simulink model "AirRefueling_Platform_ch10_WindEffect"  (R2022a)
settings: Solver=ode3  StartTime=0.0  StopTime=150  FixedStep=0.01  RelTol=1e-5  AbsTol=1e-4  EnableMultiTasking=on
InitFcn:
  | F16_Init
values from neighbouring files (symbols this model uses):
  airSpeed = 393.72    [F16_Init.m]
  alpha0 = trimAlpha*180/pi    (= 6.62393794015)    [F16_Init.m]
  altitude = 9843    [F16_Init.m]
  b_ref = 30.0    (= 30)    [F16_Init.m]
  C = [ 1,0,0,zeros(1,15) ... (first row only)    [F16_Init.m]
  C2m = [C(1,:) ... (first row only)    [F16_Init.m]
  d_f_rc = [4.45;0;-3.81]    [F16_Init.m]
  d_pr_rc = [8.2;0.45;-3.3]    [F16_Init.m]
  dLEF = 0    [F16_Init.m]
  fi_flag = 1    [F16_Init.m]
  Kc = [ ... (first row only)    [F16_Init.m]
  Ki = zeros(4,3)    [F16_Init.m]
  Kp = zeros(4,18)    [F16_Init.m]
  mass = 636.94    [F16_Init.m]
  p0_pr = p0_rc + d_pr_rc    [F16_Init.m]
  p0_rc = [-28;0;0]    [F16_Init.m]
  trim_ail = 0.00874607850103852    (= 0.00874607850104)    [F16_Init.m]
  trim_control = [trim_thrust;trim_ele;trim_ail;trim_rud]    [F16_Init.m]
  trim_ele = -2.97973164860638    (= -2.97973164861)    [F16_Init.m]
  trim_rud = 0.0680302158182712    (= 0.0680302158183)    [F16_Init.m]
  trim_state1 = [trim_state;0;0;0;0;0;0]    [F16_Init.m]
  trim_thrust = 2279.08519954656    (= 2279.08519955)    [F16_Init.m]
  visual_err = [0;0;0]    [F16_Init.m]
undefined symbols (not defined in the file or in its folder): Cdr_, dockingPoint, dtheta10, dtheta20, F, height, k_reel, kd, l0, l1, l_density, Light, m0, Mdr, MIL, N, Rdr, Rl, STD, T_reel_initial, theta10, theta20, vt0
libraries: etargetslib x22, dspnetwork x20, aerolibconvert2 x6, aerolibasang x4, simulink x2, aerolibatmos2 x2, aerolibwind2 x2, aerolibobsolete x2, sharedtransform x2, aerolibutil x2, vrlib x1, aerolibadyn x1
(part 2 of 4)

== system AirRefueling_Platform_ch10_WindEffect/3D rendering engine/SendToPX4SILIntFloat ==
  note: struct PX4SILIntFloat {
      | int checksum ;
      | int CopterID ;
      | int inSILInts [ 8 ];
      | float inSILFLoats [ 20 ];
      | }
  note: This message will be sent to PX4 DLL model's input signals inSILInts[8] and inSILFloats[20].
      | The checksum should be set to 1234567897, and the data should be sent to port 30100+(i-1)*2
  inSILInts : Inport  OutDataTypeStr=int32  PortDimensions=8
  inSILFloats : Inport  Port=2  OutDataTypeStr=single  PortDimensions=20
  CopterID : Constant  Value=10  OutDataTypeStr=Inherit: Inherit via back propagation
  Data Type Conversion1 : DataTypeConversion  OutDataTypeStr=int32  SaturateOnIntegerOverflow=off  RndMeth=Floor
  Data Type Conversion2 : DataTypeConversion  OutDataTypeStr=single  SaturateOnIntegerOverflow=off  RndMeth=Floor
  Data Type Conversion3 : DataTypeConversion  OutDataTypeStr=int32  SaturateOnIntegerOverflow=off  RndMeth=Floor
  Mux : Mux  Inputs=2
  PayLoad : etargetslib/Byte Pack  datatypes={'int32','int32','single'}  byteAlign=8
  checksum : Constant  Value=1234567897  OutDataTypeStr=Inherit: Inherit via back propagation
  PX4SILIntFloat : Outport  OutDataTypeStr=uint8  PortDimensions=120  VectorParamsAs1DForOutWhenUnconnected=off
  wires:
  inSILFloats/1 -> Data Type Conversion2/1
  inSILInts/1 -> Data Type Conversion1/1
  PayLoad/1 -> PX4SILIntFloat/1
  Data Type Conversion1/1 -> PayLoad/2
  Data Type Conversion2/1 -> PayLoad/3
  checksum/1 -> Mux/1
  Mux/1 -> Data Type Conversion3/1
  Data Type Conversion3/1 -> PayLoad/1
  CopterID/1 -> Mux/2

== system AirRefueling_Platform_ch10_WindEffect/3D rendering engine/Subsystem1 ==
  copterID : Inport  PortDimensions=1
  vehicleType : Inport  Port=2  PortDimensions=1
  PosE : Inport  Port=3  PortDimensions=3
  AngEuler : Inport  Port=4  PortDimensions=3
  VelE : Inport  Port=5  PortDimensions=3
  Clock : Clock
  Constant1 : Constant  Value=[0,0,0,0]
  Constant3 : Constant  Value=[0,0,0]
  Constant4 : Constant  Value=[0,0,0]
  Constant5 : Constant  Value=[0,0,0]
  MotorPWMs1 : Constant  Value=[1000,1000,1000,1000,0,0,0,0]
  Subsystem : Subsystem
  toUnReal : Outport  VectorParamsAs1DForOutWhenUnconnected=off
  wires:
  VelE/1 -> Subsystem/4("VelE ")
  PosE/1 -> Subsystem/5(PosE)
  vehicleType/1 -> Subsystem/2(vehicleType)
  Clock/1 -> Subsystem/3(runnedTime)
  Constant4/1 -> Subsystem/10(RateB)
  Constant5/1 -> Subsystem/11(PosGPS)
  AngEuler/1 -> Subsystem/6(AngEuler)
  Subsystem/1(toUnReal) -> toUnReal/1
  Constant3/1 -> Subsystem/9(AccB)
  Constant1/1 -> Subsystem/7(AngQuatern)
  copterID/1 -> Subsystem/1(copterID)
  MotorPWMs1/1 -> Subsystem/8(MotorRPMS)

== system AirRefueling_Platform_ch10_WindEffect/3D rendering engine/VehicleAttatchreq ==
  note: struct VehicleAttatch25 {
      | 	int checksum;//1234567892
      | 	int CopterIDs[25];
      | 	int AttatchIDs[25];
      | 	int AttatchTypes[25];//0：正常模式，1：相对位置不相对姿态，2：相对位置+偏航（不相对俯仰和滚转），3：相对位置+全姿态（俯仰滚转偏航）
      | }
  CopterIDs : Inport  PortDimensions=25
  AttatchIDs : Inport  Port=2  PortDimensions=25
  AttatchTypes : Inport  Port=3  PortDimensions=25
  Constant7 : Constant  Value=1234567892
  Data Type Conversion{,1..2,4} (4 alike) : DataTypeConversion  OutDataTypeStr=int32  SaturateOnIntegerOverflow=off  RndMeth=Floor
  PayLoad : etargetslib/Byte Pack  datatypes={'int32','int32','int32','int32'}  byteAlign=4
  Out1 : Outport  VectorParamsAs1DForOutWhenUnconnected=off
  wires:
  Data Type Conversion1/1 -> PayLoad/3
  AttatchTypes/1 -> Data Type Conversion2/1
  Data Type Conversion2/1 -> PayLoad/4
  PayLoad/1 -> Out1/1
  AttatchIDs/1 -> Data Type Conversion1/1
  Data Type Conversion/1 -> PayLoad/2
  CopterIDs/1 -> Data Type Conversion/1
  Constant7/1 -> Data Type Conversion4/1
  Data Type Conversion4/1 -> PayLoad/1

== system AirRefueling_Platform_ch10_WindEffect/3D rendering engine1/20APIWithScale ==
  note: struct Multi3DData1New {
      |        int checksum;
      | 	uint16 IDs[20];
      | 	uint16 VehileTypes[20];
      | 	float PosE[60];
      | 	float AngEuler[60];
      | 	uint16 ScaleXYZ[60];
      | }
  note: scale value * 100
  IDs : Inport  PortDimensions=20
  VehileTypes : Inport  Port=2  PortDimensions=20
  PosEs : Inport  Port=3  PortDimensions=60
  AngEulers : Inport  Port=4  PortDimensions=60
  scaleXYZ : Inport  Port=5  PortDimensions=60
  Constant7 : Constant  Value=1234567890
  Data Type Conversion : DataTypeConversion  OutDataTypeStr=uint16  SaturateOnIntegerOverflow=off  RndMeth=Floor
  Data Type Conversion1 : DataTypeConversion  OutDataTypeStr=uint16  SaturateOnIntegerOverflow=off  RndMeth=Floor
  Data Type Conversion2 : DataTypeConversion  OutDataTypeStr=single  SaturateOnIntegerOverflow=off  RndMeth=Floor
  Data Type Conversion3 : DataTypeConversion  OutDataTypeStr=single  SaturateOnIntegerOverflow=off  RndMeth=Floor
  Data Type Conversion4 : DataTypeConversion  OutDataTypeStr=uint16  SaturateOnIntegerOverflow=off  RndMeth=Floor
  Data Type Conversion5 : DataTypeConversion  OutDataTypeStr=int32  SaturateOnIntegerOverflow=off  RndMeth=Floor
  Gain : Gain  Gain=100
  PayLoad : etargetslib/Byte Pack  datatypes={'int32','uint16','uint16','single','single','uint16'}  byteAlign=4
  Saturation : Saturate  UpperLimit=655.35  LowerLimit=0.01
  Out1 : Outport  VectorParamsAs1DForOutWhenUnconnected=off
  wires:
  Data Type Conversion3/1 -> PayLoad/5
  Data Type Conversion1/1 -> PayLoad/3
  PosEs/1 -> Data Type Conversion2/1
  Data Type Conversion2/1 -> PayLoad/4
  AngEulers/1 -> Data Type Conversion3/1
  PayLoad/1 -> Out1/1
  VehileTypes/1 -> Data Type Conversion1/1
  Data Type Conversion/1 -> PayLoad/2
  IDs/1 -> Data Type Conversion/1
  scaleXYZ/1 -> Saturation/1
  Data Type Conversion4/1 -> PayLoad/6
  Saturation/1 -> Gain/1
  Gain/1 -> Data Type Conversion4/1
  Constant7/1 -> Data Type Conversion5/1
  Data Type Conversion5/1 -> PayLoad/1

== system AirRefueling_Platform_ch10_WindEffect/3D rendering engine1/20APIWithScale1 ==
  note: struct Multi3DData1New {
      |        int checksum;
      | 	uint16 IDs[20];
      | 	uint16 VehileTypes[20];
      | 	float PosE[60];
      | 	float AngEuler[60];
      | 	uint16 ScaleXYZ[60];
      | }
  note: scale value * 100
  IDs : Inport  PortDimensions=20
  VehileTypes : Inport  Port=2  PortDimensions=20
  PosEs : Inport  Port=3  PortDimensions=60
  AngEulers : Inport  Port=4  PortDimensions=60
  scaleXYZ : Inport  Port=5  PortDimensions=60
  Constant7 : Constant  Value=1234567890
  Data Type Conversion : DataTypeConversion  OutDataTypeStr=uint16  SaturateOnIntegerOverflow=off  RndMeth=Floor
  Data Type Conversion1 : DataTypeConversion  OutDataTypeStr=uint16  SaturateOnIntegerOverflow=off  RndMeth=Floor
  Data Type Conversion2 : DataTypeConversion  OutDataTypeStr=single  SaturateOnIntegerOverflow=off  RndMeth=Floor
  Data Type Conversion3 : DataTypeConversion  OutDataTypeStr=single  SaturateOnIntegerOverflow=off  RndMeth=Floor
  Data Type Conversion4 : DataTypeConversion  OutDataTypeStr=uint16  SaturateOnIntegerOverflow=off  RndMeth=Floor
  Data Type Conversion5 : DataTypeConversion  OutDataTypeStr=int32  SaturateOnIntegerOverflow=off  RndMeth=Floor
  Gain : Gain  Gain=100
  PayLoad : etargetslib/Byte Pack  datatypes={'int32','uint16','uint16','single','single','uint16'}  byteAlign=4
  Saturation : Saturate  UpperLimit=655.35  LowerLimit=0.01
  Out1 : Outport  VectorParamsAs1DForOutWhenUnconnected=off
  wires:
  Data Type Conversion3/1 -> PayLoad/5
  Data Type Conversion1/1 -> PayLoad/3
  PosEs/1 -> Data Type Conversion2/1
  Data Type Conversion2/1 -> PayLoad/4
  AngEulers/1 -> Data Type Conversion3/1
  PayLoad/1 -> Out1/1
  VehileTypes/1 -> Data Type Conversion1/1
  Data Type Conversion/1 -> PayLoad/2
  IDs/1 -> Data Type Conversion/1
  scaleXYZ/1 -> Saturation/1
  Data Type Conversion4/1 -> PayLoad/6
  Saturation/1 -> Gain/1
  Gain/1 -> Data Type Conversion4/1
  Constant7/1 -> Data Type Conversion5/1
  Data Type Conversion5/1 -> PayLoad/1

== system AirRefueling_Platform_ch10_WindEffect/3D rendering engine1/OneSimpleAPIWithScal e2 ==
  note: //输出到模拟器的数据
      | struct SOut2SimulatorSimple1 {
      | 	int checkSum;
      | 	int copterID;  //Vehicle ID
      | 	int vehicleType;  //Vehicle type
      | 	float MotorRPMSMean;
      | 	float PosE[3];   //NED vehicle position in earth frame (m)
      | 	float AngEuler[3];  //Vehicle Euler angle roll pitch yaw (rad) in x y z
      | 	float Scale[3];
      | }
  note: All acutators will use this value
  copterID : Inport  PortDimensions=1
  vehicleType : Inport  Port=2  PortDimensions=1
  PosE : Inport  Port=3  PortDimensions=3
  AngEuler : Inport  Port=4  PortDimensions=3
  ScaleXYZ : Inport  Port=5  PortDimensions=3
  Constant7 : Constant  Value=1234567890
  Data Type Conversion : DataTypeConversion  OutDataTypeStr=int32  SaturateOnIntegerOverflow=off  RndMeth=Floor
  Data Type Conversion1 : DataTypeConversion  OutDataTypeStr=single  SaturateOnIntegerOverflow=off  RndMeth=Floor
  Mux : Mux  Inputs=3
  Mux1 : Mux
  PWMs : Constant  Value=3000
  PayLoad : etargetslib/Byte Pack  datatypes={'int32','single'}  byteAlign=1
  toUnReal : Outport  VectorParamsAs1DForOutWhenUnconnected=off
  wires:
  PayLoad/1 -> toUnReal/1
  Data Type Conversion/1 -> PayLoad/1
  Data Type Conversion1/1 -> PayLoad/2
  copterID/1 -> Mux/2
  vehicleType/1 -> Mux/3
  Constant7/1 -> Mux/1
  Mux/1 -> Data Type Conversion/1
  Mux1/1 -> Data Type Conversion1/1
  PWMs/1 -> Mux1/1
  PosE/1 -> Mux1/2
  AngEuler/1 -> Mux1/3
  ScaleXYZ/1 -> Mux1/4

== system AirRefueling_Platform_ch10_WindEffect/3D rendering engine1/OneSimpleAPIWithScale1 ==
  note: //输出到模拟器的数据
      | struct SOut2SimulatorSimple1 {
      | 	int checkSum;
      | 	int copterID;  //Vehicle ID
      | 	int vehicleType;  //Vehicle type
      | 	float MotorRPMSMean;
      | 	float PosE[3];   //NED vehicle position in earth frame (m)
      | 	float AngEuler[3];  //Vehicle Euler angle roll pitch yaw (rad) in x y z
      | 	float Scale[3];
      | }
  note: All acutators will use this value
  copterID : Inport  PortDimensions=1
  vehicleType : Inport  Port=2  PortDimensions=1
  PosE : Inport  Port=3  PortDimensions=3
  AngEuler : Inport  Port=4  PortDimensions=3
  ScaleXYZ : Inport  Port=5  PortDimensions=3
  Constant7 : Constant  Value=1234567890
  Data Type Conversion : DataTypeConversion  OutDataTypeStr=int32  SaturateOnIntegerOverflow=off  RndMeth=Floor
  Data Type Conversion1 : DataTypeConversion  OutDataTypeStr=single  SaturateOnIntegerOverflow=off  RndMeth=Floor
  Mux : Mux  Inputs=3
  Mux1 : Mux
  PWMs : Constant  Value=3000
  PayLoad : etargetslib/Byte Pack  datatypes={'int32','single'}  byteAlign=1
  toUnReal : Outport  VectorParamsAs1DForOutWhenUnconnected=off
  wires:
  PayLoad/1 -> toUnReal/1
  Data Type Conversion/1 -> PayLoad/1
  Data Type Conversion1/1 -> PayLoad/2
  copterID/1 -> Mux/2
  vehicleType/1 -> Mux/3
  Constant7/1 -> Mux/1
  Mux/1 -> Data Type Conversion/1
  Mux1/1 -> Data Type Conversion1/1
  PWMs/1 -> Mux1/1
  PosE/1 -> Mux1/2
  AngEuler/1 -> Mux1/3
  ScaleXYZ/1 -> Mux1/4

== system AirRefueling_Platform_ch10_WindEffect/3D rendering engine1/OneSimpleAPIWithScale3 ==
  note: All acutators will use this value
  note: //输出到模拟器的数据
      | struct SOut2SimulatorSimple1 {
      | 	int checkSum;
      | 	int copterID;  //Vehicle ID
      | 	int vehicleType;  //Vehicle type
      | 	float MotorRPMSMean;
      | 	float PosE[3];   //NED vehicle position in earth frame (m)
      | 	float AngEuler[3];  //Vehicle Euler angle roll pitch yaw (rad) in x y z
      | 	float Scale[3];
      | }
  copterID : Inport  PortDimensions=1
  vehicleType : Inport  Port=2  PortDimensions=1
  PosE : Inport  Port=3  PortDimensions=3
  AngEuler : Inport  Port=4  PortDimensions=3
  ScaleXYZ : Inport  Port=5  PortDimensions=3
  Constant7 : Constant  Value=1234567890
  Data Type Conversion : DataTypeConversion  OutDataTypeStr=int32  SaturateOnIntegerOverflow=off  RndMeth=Floor
  Data Type Conversion1 : DataTypeConversion  OutDataTypeStr=single  SaturateOnIntegerOverflow=off  RndMeth=Floor
  Mux : Mux  Inputs=3
  Mux1 : Mux
  PWMs : Constant  Value=3000
  PayLoad : etargetslib/Byte Pack  datatypes={'int32','single'}  byteAlign=1
  toUnReal : Outport  VectorParamsAs1DForOutWhenUnconnected=off
  wires:
  ScaleXYZ/1 -> Mux1/4
  AngEuler/1 -> Mux1/3
  PosE/1 -> Mux1/2
  PWMs/1 -> Mux1/1
  Mux1/1 -> Data Type Conversion1/1
  Mux/1 -> Data Type Conversion/1
  Constant7/1 -> Mux/1
  vehicleType/1 -> Mux/3
  copterID/1 -> Mux/2
  Data Type Conversion1/1 -> PayLoad/2
  Data Type Conversion/1 -> PayLoad/1
  PayLoad/1 -> toUnReal/1

== system AirRefueling_Platform_ch10_WindEffect/3D rendering engine1/OneSimpleAPIWithScale4 ==
  note: All acutators will use this value
  note: //输出到模拟器的数据
      | struct SOut2SimulatorSimple1 {
      | 	int checkSum;
      | 	int copterID;  //Vehicle ID
      | 	int vehicleType;  //Vehicle type
      | 	float MotorRPMSMean;
      | 	float PosE[3];   //NED vehicle position in earth frame (m)
      | 	float AngEuler[3];  //Vehicle Euler angle roll pitch yaw (rad) in x y z
      | 	float Scale[3];
      | }
  copterID : Inport  PortDimensions=1
  vehicleType : Inport  Port=2  PortDimensions=1
  PosE : Inport  Port=3  PortDimensions=3
  AngEuler : Inport  Port=4  PortDimensions=3
  ScaleXYZ : Inport  Port=5  PortDimensions=3
  Constant7 : Constant  Value=1234567890
  Data Type Conversion : DataTypeConversion  OutDataTypeStr=int32  SaturateOnIntegerOverflow=off  RndMeth=Floor
  Data Type Conversion1 : DataTypeConversion  OutDataTypeStr=single  SaturateOnIntegerOverflow=off  RndMeth=Floor
  Mux : Mux  Inputs=3
  Mux1 : Mux
  PWMs : Constant  Value=3000
  PayLoad : etargetslib/Byte Pack  datatypes={'int32','single'}  byteAlign=1
  toUnReal : Outport  VectorParamsAs1DForOutWhenUnconnected=off
  wires:
  ScaleXYZ/1 -> Mux1/4
  AngEuler/1 -> Mux1/3
  PosE/1 -> Mux1/2
  PWMs/1 -> Mux1/1
  Mux1/1 -> Data Type Conversion1/1
  Mux/1 -> Data Type Conversion/1
  Constant7/1 -> Mux/1
  vehicleType/1 -> Mux/3
  copterID/1 -> Mux/2
  Data Type Conversion1/1 -> PayLoad/2
  Data Type Conversion/1 -> PayLoad/1
  PayLoad/1 -> toUnReal/1

== system AirRefueling_Platform_ch10_WindEffect/3D rendering engine1/OneSimpleAPIWithScale5 ==
  note: //输出到模拟器的数据
      | struct SOut2SimulatorSimple1 {
      | 	int checkSum;
      | 	int copterID;  //Vehicle ID
      | 	int vehicleType;  //Vehicle type
      | 	float MotorRPMSMean;
      | 	float PosE[3];   //NED vehicle position in earth frame (m)
      | 	float AngEuler[3];  //Vehicle Euler angle roll pitch yaw (rad) in x y z
      | 	float Scale[3];
      | }
  note: All acutators will use this value
  copterID : Inport  PortDimensions=1
  vehicleType : Inport  Port=2  PortDimensions=1
  PosE : Inport  Port=3  PortDimensions=3
  AngEuler : Inport  Port=4  PortDimensions=3
  ScaleXYZ : Inport  Port=5  PortDimensions=3
  Constant7 : Constant  Value=1234567890
  Data Type Conversion : DataTypeConversion  OutDataTypeStr=int32  SaturateOnIntegerOverflow=off  RndMeth=Floor
  Data Type Conversion1 : DataTypeConversion  OutDataTypeStr=single  SaturateOnIntegerOverflow=off  RndMeth=Floor
  Mux : Mux  Inputs=3
  Mux1 : Mux
  PWMs : Constant  Value=3000
  PayLoad : etargetslib/Byte Pack  datatypes={'int32','single'}  byteAlign=1
  toUnReal : Outport  VectorParamsAs1DForOutWhenUnconnected=off
  wires:
  PayLoad/1 -> toUnReal/1
  Data Type Conversion/1 -> PayLoad/1
  Data Type Conversion1/1 -> PayLoad/2
  copterID/1 -> Mux/2
  vehicleType/1 -> Mux/3
  Constant7/1 -> Mux/1
  Mux/1 -> Data Type Conversion/1
  Mux1/1 -> Data Type Conversion1/1
  PWMs/1 -> Mux1/1
  PosE/1 -> Mux1/2
  AngEuler/1 -> Mux1/3
  ScaleXYZ/1 -> Mux1/4

== system AirRefueling_Platform_ch10_WindEffect/3D rendering engine1/SendToPX4SILIntFloat ==
  note: struct PX4SILIntFloat {
      | int checksum ;
      | int CopterID ;
      | int inSILInts [ 8 ];
      | float inSILFLoats [ 20 ];
      | }
  note: This message will be sent to PX4 DLL model's input signals inSILInts[8] and inSILFloats[20].
      | The checksum should be set to 1234567897, and the data should be sent to port 30100+(i-1)*2
  inSILInts : Inport  OutDataTypeStr=int32  PortDimensions=8
  inSILFloats : Inport  Port=2  OutDataTypeStr=single  PortDimensions=20
  CopterID : Constant  Value=10  OutDataTypeStr=Inherit: Inherit via back propagation
  Data Type Conversion1 : DataTypeConversion  OutDataTypeStr=int32  SaturateOnIntegerOverflow=off  RndMeth=Floor
  Data Type Conversion2 : DataTypeConversion  OutDataTypeStr=single  SaturateOnIntegerOverflow=off  RndMeth=Floor
  Data Type Conversion3 : DataTypeConversion  OutDataTypeStr=int32  SaturateOnIntegerOverflow=off  RndMeth=Floor
  Mux : Mux  Inputs=2
  PayLoad : etargetslib/Byte Pack  datatypes={'int32','int32','single'}  byteAlign=8
  checksum : Constant  Value=1234567897  OutDataTypeStr=Inherit: Inherit via back propagation
  PX4SILIntFloat : Outport  OutDataTypeStr=uint8  PortDimensions=120  VectorParamsAs1DForOutWhenUnconnected=off
  wires:
  inSILFloats/1 -> Data Type Conversion2/1
  inSILInts/1 -> Data Type Conversion1/1
  PayLoad/1 -> PX4SILIntFloat/1
  Data Type Conversion1/1 -> PayLoad/2
  Data Type Conversion2/1 -> PayLoad/3
  checksum/1 -> Mux/1
  Mux/1 -> Data Type Conversion3/1
  Data Type Conversion3/1 -> PayLoad/1
  CopterID/1 -> Mux/2

== system AirRefueling_Platform_ch10_WindEffect/3D rendering engine1/Subsystem1 ==
  copterID : Inport  PortDimensions=1
  vehicleType : Inport  Port=2  PortDimensions=1
  PosE : Inport  Port=3  PortDimensions=3
  AngEuler : Inport  Port=4  PortDimensions=3
  VelE : Inport  Port=5  PortDimensions=3
  Clock : Clock
  Constant1 : Constant  Value=[0,0,0,0]
  Constant3 : Constant  Value=[0,0,0]
  Constant4 : Constant  Value=[0,0,0]
  Constant5 : Constant  Value=[0,0,0]
  MotorPWMs1 : Constant  Value=[1000,1000,1000,1000,0,0,0,0]
  Subsystem : Subsystem
  toUnReal : Outport  VectorParamsAs1DForOutWhenUnconnected=off
  wires:
  VelE/1 -> Subsystem/4("VelE ")
  PosE/1 -> Subsystem/5(PosE)
  vehicleType/1 -> Subsystem/2(vehicleType)
  Clock/1 -> Subsystem/3(runnedTime)
  Constant4/1 -> Subsystem/10(RateB)
  Constant5/1 -> Subsystem/11(PosGPS)
  AngEuler/1 -> Subsystem/6(AngEuler)
  Subsystem/1(toUnReal) -> toUnReal/1
  Constant3/1 -> Subsystem/9(AccB)
  Constant1/1 -> Subsystem/7(AngQuatern)
  copterID/1 -> Subsystem/1(copterID)
  MotorPWMs1/1 -> Subsystem/8(MotorRPMS)

== system AirRefueling_Platform_ch10_WindEffect/3D rendering engine1/VehicleAttatchreq ==
  note: struct VehicleAttatch25 {
      | 	int checksum;//1234567892
      | 	int CopterIDs[25];
      | 	int AttatchIDs[25];
      | 	int AttatchTypes[25];//0：正常模式，1：相对位置不相对姿态，2：相对位置+偏航（不相对俯仰和滚转），3：相对位置+全姿态（俯仰滚转偏航）
      | }
  CopterIDs : Inport  PortDimensions=25
  AttatchIDs : Inport  Port=2  PortDimensions=25
  AttatchTypes : Inport  Port=3  PortDimensions=25
  Constant7 : Constant  Value=1234567892
  Data Type Conversion{,1..2,4} (4 alike) : DataTypeConversion  OutDataTypeStr=int32  SaturateOnIntegerOverflow=off  RndMeth=Floor
  PayLoad : etargetslib/Byte Pack  datatypes={'int32','int32','int32','int32'}  byteAlign=4
  Out1 : Outport  VectorParamsAs1DForOutWhenUnconnected=off
  wires:
  Data Type Conversion1/1 -> PayLoad/3
  AttatchTypes/1 -> Data Type Conversion2/1
  Data Type Conversion2/1 -> PayLoad/4
  PayLoad/1 -> Out1/1
  AttatchIDs/1 -> Data Type Conversion1/1
  Data Type Conversion/1 -> PayLoad/2
  CopterIDs/1 -> Data Type Conversion/1
  Constant7/1 -> Data Type Conversion4/1
  Data Type Conversion4/1 -> PayLoad/1

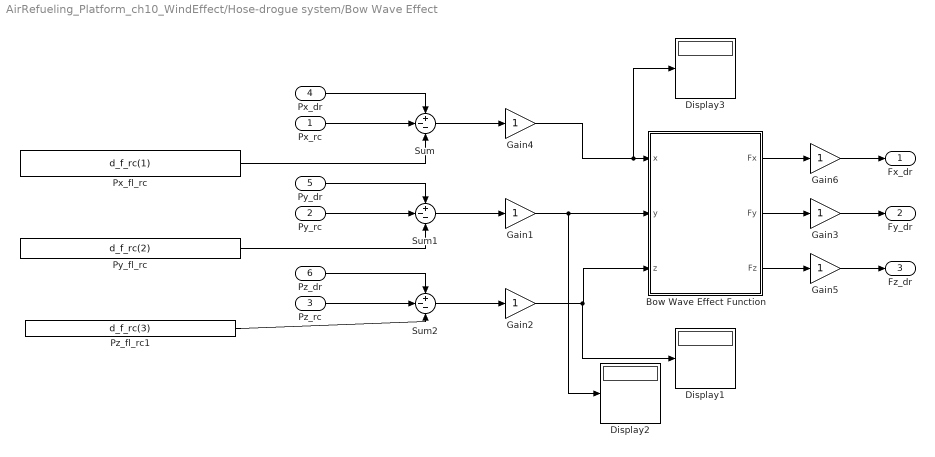
== system AirRefueling_Platform_ch10_WindEffect/Hose-drogue system/Bow Wave Effect ==
  Px_rc : Inport
  Py_rc : Inport  Port=2
  Pz_rc : Inport  Port=3
  Px_dr : Inport  Port=4
  Py_dr : Inport  Port=5
  Pz_dr : Inport  Port=6
  Bow Wave Effect Function : MATLAB Function  TreatAsAtomicUnit=on
  Display1 : Display
  Display2 : Display
  Display3 : Display
  Gain{1..6} (6 alike) : Gain
  Px_fl_rc : Constant  Value=d_f_rc(1)
  Py_fl_rc : Constant  Value=d_f_rc(2)
  Pz_fl_rc1 : Constant  Value=d_f_rc(3)
  Sum : Sum  Inputs=+--
  Sum1 : Sum  Inputs=+--
  Sum2 : Sum  Inputs=+--
  Fx_dr : Outport
  Fy_dr : Outport  Port=2
  Fz_dr : Outport  Port=3
  wires:
  Sum2/1 -> Gain2/1
  Sum1/1 -> Gain1/1
  Bow Wave Effect Function/3(Fz) -> Gain5/1
  Bow Wave Effect Function/2(Fy) -> Gain3/1
  Bow Wave Effect Function/1(Fx) -> Gain6/1
  Gain6/1 -> Fx_dr/1
  Gain5/1 -> Fz_dr/1
  Gain3/1 -> Fy_dr/1
  Gain2/1 -> Display1/1, Bow Wave Effect Function/3(z)
  Gain1/1 -> Display2/1, Bow Wave Effect Function/2(y)
  Gain4/1 -> Display3/1, Bow Wave Effect Function/1(x)
  Pz_dr/1 -> Sum2/1
  Pz_fl_rc1/1 -> Sum2/3
  Pz_rc/1 -> Sum2/2
  Py_fl_rc/1 -> Sum1/3
  Py_dr/1 -> Sum1/1
  Py_rc/1 -> Sum1/2
  Px_dr/1 -> Sum/1
  Px_fl_rc/1 -> Sum/3
  Px_rc/1 -> Sum/2
  Sum/1 -> Gain4/1

== system AirRefueling_Platform_ch10_WindEffect/Hose-drogue system/Collision Detection ==
  note: 这里的结果和发送坐标相同
  note: 相对距离
  note: 椎管的位置
  note: 椎管的速度
  note: 相对速度
  Pos_rc2tx : Inport
  Pos_dr : Inport  Port=2
  Constant : Constant  Value=d_pr_rc
  Constant1 : Constant  Value=Mdr
  Derivative : Derivative
  Derivative1 : Derivative
  Display1 : Display
  Display6 : Display
  MATLAB Function1 : MATLAB Function  TreatAsAtomicUnit=on
  Scope1 : Scope
  Scope2 : Scope
  Scope3 : Scope
  Sum1 : Sum  Inputs=|+-+
  Sum2 : Sum  Inputs=|++
  Sum3 : Sum  Inputs=|+-
  Sum5 : Sum  Inputs=|++
  drogue_delta_pos : Constant  Value=[0,0,0.04]
  修正数据让对接时误差为0 : Constant  Value=visual_err
  y : Outport
  wires:
  MATLAB Function1/1(F) -> Scope3/1, y/1
  Constant/1 -> Sum2/1
  Derivative/1 -> Sum3/1, MATLAB Function1/2(V_pr)
  Derivative1/1 -> Sum3/2, MATLAB Function1/4(V_dr)
  Constant1/1 -> MATLAB Function1/5(Mdr)
  Sum1/1 -> Display6/1, Scope1/1
  Sum3/1 -> Display1/1, Scope2/1
  Sum2/1 -> Derivative/1, Sum1/2, MATLAB Function1/1(Pos_pr)
  Sum5/1 -> Sum1/3, MATLAB Function1/3(Pos_dr), Derivative1/1
  Pos_dr/1 -> Sum5/1
  drogue_delta_pos/1 -> Sum5/2
  Pos_rc2tx/1 -> Sum2/2
  修正数据让对接时误差为0/1 -> MATLAB Function1/6(visual_err), Sum1/1

== system AirRefueling_Platform_ch10_WindEffect/Hose-drogue system/DRdynamics ==
  Fx_dr : Inport
  Fy_dr : Inport  Port=2
  Fz_dr : Inport  Port=3
  Tanker_States : Inport  Port=4
  Demux : Demux  Outputs=3
  Demux1 : Demux  Outputs=3
  HDU : Subsystem
  Hose-Drogue1 : Subsystem
  Memory : Memory  InitialCondition=T_reel_initial
  Mux1 : Mux  Inputs=3
  Scope1 : Scope
  Scope2 : Scope
  Scope38 : Scope
  To Workspace1 : ToWorkspace  VariableName=dl_1  SampleTime=-1
  To Workspace2 : ToWorkspace  VariableName=ddl_1  SampleTime=-1
  To Workspace3 : ToWorkspace  VariableName=T_hose  SampleTime=-1
  length2 : Constant  Value=zeros(3,N)
  Pxdr_tk : Outport
  Pydr_tk : Outport  Port=2
  Pzdr_tk : Outport  Port=3
  plink : Outport  Port=4
  wires:
  Demux1/1 -> Hose-Drogue1/1(pt)
  Demux1/2 -> Hose-Drogue1/2(vt)
  Demux1/3 -> Hose-Drogue1/3(at)
  length2/1 -> Hose-Drogue1/4(w)
  Hose-Drogue1/2(t) -> Scope38/1, Memory/1, To Workspace3/1
  Memory/1 -> HDU/1(t_hose)
  HDU/1(l_1) -> Hose-Drogue1/5(link length)
  HDU/3(ddl_1) -> Hose-Drogue1/7(DD link length), Scope2/1, To Workspace2/1
  Hose-Drogue1/1(p link) -> plink/1
  Mux1/1 -> Hose-Drogue1/8(Fb)
  Fx_dr/1 -> Mux1/1
  Fy_dr/1 -> Mux1/2
  Fz_dr/1 -> Mux1/3
  Hose-Drogue1/3(pdr) -> Demux/1
  Demux/1 -> Pxdr_tk/1
  Demux/2 -> Pydr_tk/1
  Demux/3 -> Pzdr_tk/1
  Tanker_States/1 -> Demux1/1
  HDU/2(dl_1) -> To Workspace1/1, Scope1/1, Hose-Drogue1/6(D link length)

== system AirRefueling_Platform_ch10_WindEffect/Receiver system/Controller ==
  note: u
  note: -kx
  note: u'
  note: e
  note: 跟踪控制
      | 设计反馈矩阵 Ki 使得误差 e 收敛为0
  note: x'=Ax+Bu
      | 增稳控制 u = Kp * x
      | 设计反馈矩阵 Kp 配置极点
  F16State : Inport
  Pos_Demand : Inport  Port=2
  C : Gain  Gain=C  Multiplication=Matrix(K*u) (u vector)
  Constant : Constant  Value=trim_control
  Demux : Demux
  Demux1 : Demux  Outputs=3
  Display : Display
  Gain : Gain  Gain=1000
  Gain1 : Gain  Gain=[1,0,0;0,0,-1;0,1,0]  Multiplication=Matrix(K*u) (u vector)
  Integrator : Integrator
  Integrator1 : Integrator
  Integrator2 : Integrator
  Ki : Gain  Gain=Ki  Multiplication=Matrix(K*u) (u vector)
  Kp : Gain  Gain=Kp  Multiplication=Matrix(K*u) (u vector)
  Length Conversion : aerolibconvert2/Length Conversion  IU=m  OU=ft
  Mux : Mux
  Mux3 : Mux  Inputs=3
  Saturation : Saturate  UpperLimit=15  LowerLimit=-15
  Sum : Sum  Inputs=|++
  Sum2 : Sum  Inputs=|+-
  Sum3 : Sum  Inputs=+|-
  U : Outport
  wires:
  Sum2/1 -> Demux1/1
  C/1 -> Sum2/2
  Mux3/1 -> Ki/1
  Demux1/2 -> Integrator1/1
  F16State/1 -> Display/1, Kp/1, C/1
  Integrator1/1 -> Mux3/2
  Integrator/1 -> Mux3/1
  Demux1/3 -> Integrator2/1
  Integrator2/1 -> Mux3/3
  Length Conversion/1 -> Sum2/1
  Demux1/1 -> Saturation/1
  Ki/1 -> Sum3/1
  Kp/1 -> Sum3/2
  Sum3/1 -> Demux/1
  Saturation/1 -> Integrator/1
  Demux/2 -> Mux/2
  Demux/3 -> Mux/3
  Demux/4 -> Mux/4
  Demux/1 -> Gain/1
  Gain/1 -> Mux/1
  Pos_Demand/1 -> Gain1/1
  Gain1/1 -> Length Conversion/1
  Constant/1 -> Sum/2
  Mux/1 -> Sum/1
  Sum/1 -> U/1

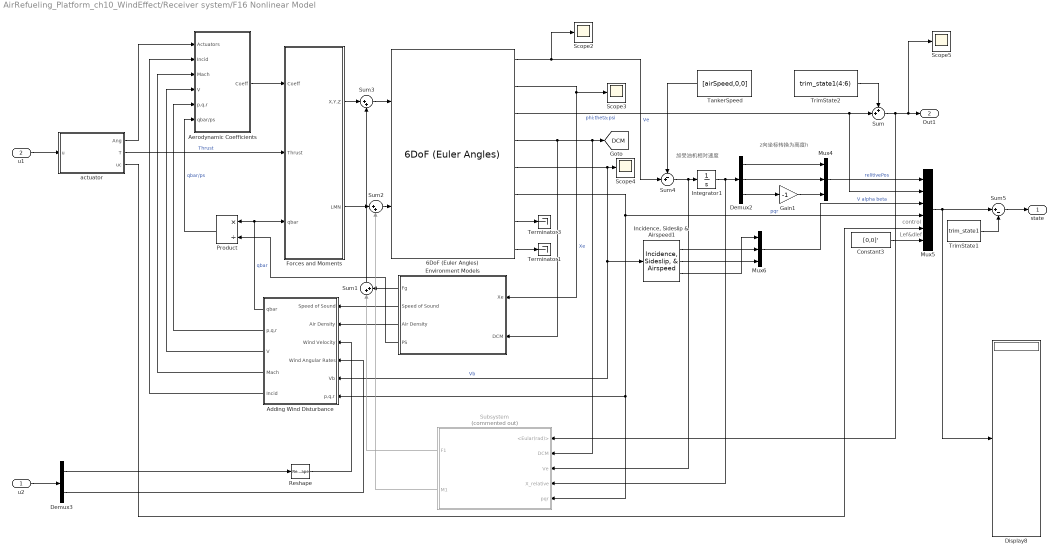
== system AirRefueling_Platform_ch10_WindEffect/Receiver system/F16 Nonlinear Model ==
  note: 加受油机相对速度
  note: z向坐标转换为高度h
  note: Lef&dlef
  note: control
  u2 : Inport
  u1 : Inport  Port=2
  6DoF (Euler Angles) : aerolibobsolete/6DoF (Euler Angles)  units=English (Velocity in ft/s)  mtype=Fixed  rep=Euler Angles  xme_0=xyz_0  Vm_0=uvw_0  eul_0=Euler_0  pm_0=pqr_0  mass_0=mass  mass_e=0.5  mass_f=2.0  inertia=Inertia  inertia_e=eye(3)  inertia_f=2*eye(3)  k_quat=1.0
      settings: SourceProductBaseCode=AE
  Adding Wind Disturbance : Subsystem
  Aerodynamic Coefficients : Subsystem
  Constant3 : Constant  Value=[0,0]'
  Demux2 : Demux  Outputs=3
  Demux3 : Demux  Outputs=2
  Display8 : Display
  Environment Models : Subsystem
  Forces and Moments : Subsystem
  Gain1 : Gain  Gain=-1
  "Incidence, Sideslip & Airspeed1" : aerolibasang/Incidence, Sideslip, & Airspeed
  Integrator1 : Integrator
  Mux4 : Mux  Inputs=3
  Mux5 : Mux  Inputs=6
  Mux6 : Mux  Inputs=3
  Product : Product  Inputs=*/  InputSameDT=on  SaturateOnIntegerOverflow=on  OutDataTypeStr=Inherit: Same as first input
  Reshape : Reshape
  Scope{2..5} (4 alike) : Scope
  Subsystem : Subsystem  Commented=on
  Sum : Sum  Inputs=++|
  Sum1 : Sum  Inputs=|++  InputSameDT=on  SaturateOnIntegerOverflow=on  OutDataTypeStr=Inherit: Same as first input
  Sum2 : Sum  Inputs=|++  InputSameDT=on  SaturateOnIntegerOverflow=on  OutDataTypeStr=Inherit: Same as first input
  Sum3 : Sum  Inputs=|++  InputSameDT=on  SaturateOnIntegerOverflow=on  OutDataTypeStr=Inherit: Same as first input
  Sum4 : Sum  Inputs=-+|
  Sum5 : Sum  Inputs=|+-
  TankerSpeed : Constant  Value=[airSpeed,0,0]
  Terminator1 : Terminator
  Terminator3 : Terminator
  TrimState1 : Constant  Value=trim_state1
  TrimState2 : Constant  Value=trim_state1(4:6)
  actuator : Subsystem
  state : Outport
  Out1 : Outport  Port=2
  tag scope: DCM=global
  wires:
  6DoF (Euler Angles)/8 -> Terminator1/1
  6DoF (Euler Angles)/7 -> Terminator3/1
  Adding Wind Disturbance/5(Incid) -> Aerodynamic Coefficients/2(Incid)
  Aerodynamic Coefficients/1(Coeff) -> Forces and Moments/1(Coeff)
  Environment Models/2(Speed of Sound) -> Adding Wind Disturbance/1(Speed of Sound)
  Environment Models/3(Air Density) -> Adding Wind Disturbance/2(Air Density)
  Adding Wind Disturbance/1(qbar) -> Forces and Moments/3(qbar), Product/1  "qbar"
  Forces and Moments/1(X,Y,Z) -> Sum3/1
  Sum3/1 -> 6DoF (Euler Angles)/1
  Adding Wind Disturbance/3(V) -> Aerodynamic Coefficients/4(V)
  Adding Wind Disturbance/4(Mach) -> Aerodynamic Coefficients/3(Mach)
  Adding Wind Disturbance/2("p,q,r ") -> Aerodynamic Coefficients/5(p,q,r)
  Environment Models/4(PS) -> Product/2
  Product/1 -> Aerodynamic Coefficients/6(qbar/ps)  "qbar/ps"
  u1/1 -> actuator/1(u)
  actuator/2(T) -> Forces and Moments/2(Thrust)  "Thrust"
  actuator/1(Ang) -> Aerodynamic Coefficients/1(Actuators)
  6DoF (Euler Angles)/3 -> Mux5/2, Sum/2  "phi;theta;psi"
  "Incidence, Sideslip & Airspeed1"/1 -> Mux6/2
  "Incidence, Sideslip & Airspeed1"/2 -> Mux6/3
  Mux6/1 -> Mux5/3  "V alpha beta"
  "Incidence, Sideslip & Airspeed1"/3 -> Mux6/1
  6DoF (Euler Angles)/6 -> Subsystem/5(pqr), Adding Wind Disturbance/6(p,q,r), Mux5/4  "pqr"
  6DoF (Euler Angles)/5 -> Scope4/1, Adding Wind Disturbance/5(Vb), "Incidence, Sideslip & Airspeed1"/1  "Vb"
  Mux5/1 -> Display8/1, Sum5/1
  TrimState1/1 -> Sum5/2
  Sum5/1 -> state/1
  actuator/3(uc) -> Mux5/5
  Constant3/1 -> Mux5/6
  Demux2/2 -> Mux4/2
  Demux2/3 -> Gain1/1
  Mux4/1 -> Mux5/1  "relitivePos"
  Demux2/1 -> Mux4/1
  Gain1/1 -> Mux4/3
  Sum4/1 -> Subsystem/3(Ve), Integrator1/1
  Integrator1/1 -> Subsystem/4(X_relative), Demux2/1
  6DoF (Euler Angles)/2 -> Scope3/1, Environment Models/1(Xe)  "Xe"
  u2/1 -> Demux3/1
  Reshape/1 -> Adding Wind Disturbance/3(Wind Velocity)
  Demux3/1 -> Reshape/1
  Demux3/2 -> Adding Wind Disturbance/4(Wind Angular Rates)
  TrimState2/1 -> Sum/1
  6DoF (Euler Angles)/1 -> Scope2/1, Sum4/2  "Ve"
  TankerSpeed/1 -> Sum4/1
  Sum/1 -> Subsystem/1(<Eular(rad)>), Scope5/1, Out1/1
  6DoF (Euler Angles)/4 -> Environment Models/2(DCM), [DCM], Subsystem/2(DCM)
  Environment Models/1(Fg) -> Sum1/2
  Subsystem/1(F1) -> Sum1/1
  Sum1/1 -> Sum3/2
  Forces and Moments/2(LMN) -> Sum2/1
  Sum2/1 -> 6DoF (Euler Angles)/2
  Subsystem/2(M1) -> Sum2/2

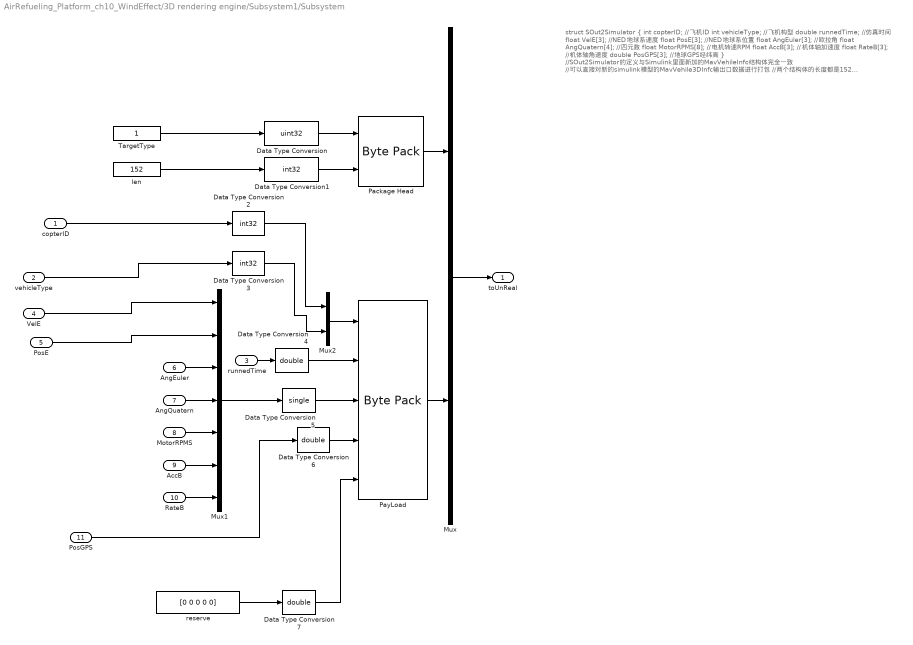
== system AirRefueling_Platform_ch10_WindEffect/3D rendering engine/Subsystem1/Subsystem ==
  note: struct SOut2Simulator
      | {
      | int copterID; //飞机ID
      | int vehicleType; //飞机构型
      | double runnedTime; //仿真时间
      | float VelE[3]; //NED地球系速度
      | float PosE[3]; //NED地球系位置
      | float AngEuler[3]; //欧拉角
      | float AngQuatern[4]; //四元数
      | float MotorRPMS[8]; //电机转速RPM
      | float AccB[3]; //机体轴加速度
      | float RateB[3]; //机体轴角速度
      | double PosGPS[3]; //地球GPS经纬高
      | }
      |
      | //SOut2Simulator的定义与Simulink里面新加的MavVehileInfo结构体完全一致
      | //可以直接对新的simulink模型的MavVehile3DInfo输出口数据进行打包
      | //两个结构体的长度都是152
      | sizeof(SOut2Simulator) = sizeof(MavVehileInfo) = 152
      |
      | 打包封装的结构体为
      | typedef struct _netDataShort
      | {
      | TargetType tg; //这里目前随便填，写1即可 uint32
      | int len; //这个长度为传输结构体长度，目前是152
      | char payload[192]; //这里面前152位存放了SOut2Simulator结构体数据，后面的40位保留
      | }netDataShort;
      |
      | //UDP包的总长度为200
      | sizeof(netDataShort) = 200
      |
      | //发送的UDP端口号为：20010
  copterID : Inport  PortDimensions=1
  vehicleType : Inport  Port=2  PortDimensions=1
  runnedTime : Inport  Port=3  PortDimensions=1
  "VelE " : Inport  Port=4  PortDimensions=3
  PosE : Inport  Port=5  PortDimensions=3
  AngEuler : Inport  Port=6  PortDimensions=3
  AngQuatern : Inport  Port=7  PortDimensions=4
  MotorRPMS : Inport  Port=8  PortDimensions=8
  AccB : Inport  Port=9  PortDimensions=3
  RateB : Inport  Port=10  PortDimensions=3
  PosGPS : Inport  Port=11  PortDimensions=3
  Data Type Conversion : DataTypeConversion  OutDataTypeStr=uint32  SaturateOnIntegerOverflow=off  RndMeth=Floor
  Data Type Conversion1 : DataTypeConversion  OutDataTypeStr=int32  SaturateOnIntegerOverflow=off  RndMeth=Floor
  Data Type Conversion2 : DataTypeConversion  OutDataTypeStr=int32  SaturateOnIntegerOverflow=off  RndMeth=Floor
  Data Type Conversion3 : DataTypeConversion  OutDataTypeStr=int32  SaturateOnIntegerOverflow=off  RndMeth=Floor
  Data Type Conversion4 : DataTypeConversion  OutDataTypeStr=double  SaturateOnIntegerOverflow=off  RndMeth=Floor
  Data Type Conversion5 : DataTypeConversion  OutDataTypeStr=single  SaturateOnIntegerOverflow=off  RndMeth=Floor
  Data Type Conversion6 : DataTypeConversion  OutDataTypeStr=double  SaturateOnIntegerOverflow=off  RndMeth=Floor
  Data Type Conversion7 : DataTypeConversion  OutDataTypeStr=double  SaturateOnIntegerOverflow=off  RndMeth=Floor
  Mux : Mux  Inputs=2
  Mux1 : Mux  Inputs=7
  Mux2 : Mux  Inputs=2
  Package Head : etargetslib/Byte Pack  datatypes={'uint32','int32'}  byteAlign=4
  PayLoad : etargetslib/Byte Pack  datatypes={'int32','double','single','double','double'}  byteAlign=8
  TargetType : Constant  OutDataTypeStr=Inherit: Inherit via back propagation
  len : Constant  Value=152  OutDataTypeStr=Inherit: Inherit via back propagation
  reserve : Constant  Value=[0 0 0 0 0]  OutDataTypeStr=double
  toUnReal : Outport  VectorParamsAs1DForOutWhenUnconnected=off
  wires:
  runnedTime/1 -> Data Type Conversion4/1
  RateB/1 -> Mux1/7
  PayLoad/1 -> Mux/2
  "VelE "/1 -> Mux1/1
  Mux1/1 -> Data Type Conversion5/1
  PosGPS/1 -> Data Type Conversion6/1
  Package Head/1 -> Mux/1
  AccB/1 -> Mux1/6
  Mux/1 -> toUnReal/1
  MotorRPMS/1 -> Mux1/5
  AngQuatern/1 -> Mux1/4
  copterID/1 -> Data Type Conversion2/1
  len/1 -> Data Type Conversion1/1
  vehicleType/1 -> Data Type Conversion3/1
  PosE/1 -> Mux1/2
  TargetType/1 -> Data Type Conversion/1
  reserve/1 -> Data Type Conversion7/1
  Mux2/1 -> PayLoad/1
  AngEuler/1 -> Mux1/3
  Data Type Conversion5/1 -> PayLoad/3
  Data Type Conversion2/1 -> Mux2/1
  Data Type Conversion1/1 -> Package Head/2
  Data Type Conversion6/1 -> PayLoad/4
  Data Type Conversion/1 -> Package Head/1
  Data Type Conversion3/1 -> Mux2/2
  Data Type Conversion4/1 -> PayLoad/2
  Data Type Conversion7/1 -> PayLoad/5

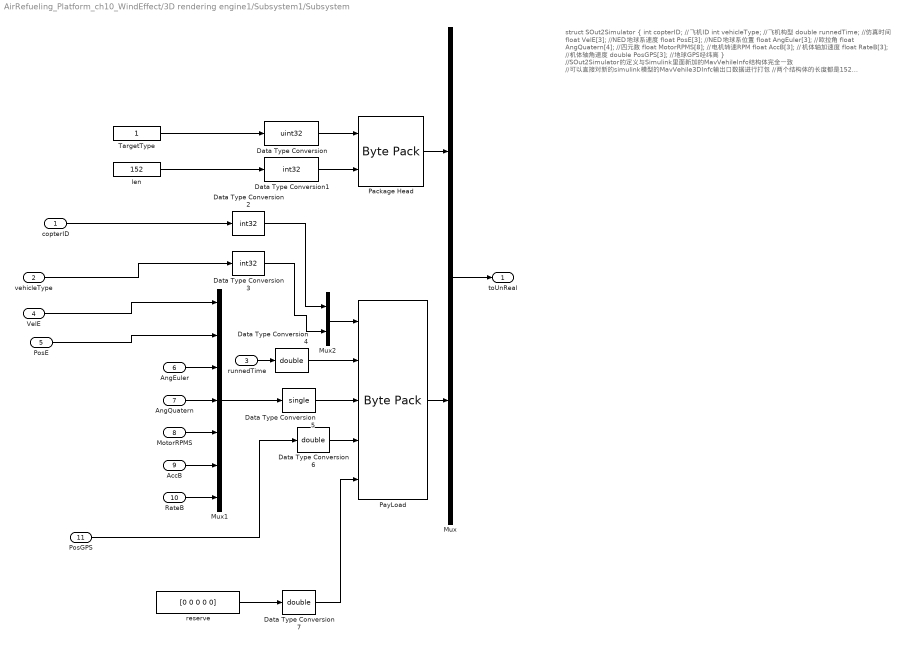
== system AirRefueling_Platform_ch10_WindEffect/3D rendering engine1/Subsystem1/Subsystem ==
  note: struct SOut2Simulator
      | {
      | int copterID; //飞机ID
      | int vehicleType; //飞机构型
      | double runnedTime; //仿真时间
      | float VelE[3]; //NED地球系速度
      | float PosE[3]; //NED地球系位置
      | float AngEuler[3]; //欧拉角
      | float AngQuatern[4]; //四元数
      | float MotorRPMS[8]; //电机转速RPM
      | float AccB[3]; //机体轴加速度
      | float RateB[3]; //机体轴角速度
      | double PosGPS[3]; //地球GPS经纬高
      | }
      |
      | //SOut2Simulator的定义与Simulink里面新加的MavVehileInfo结构体完全一致
      | //可以直接对新的simulink模型的MavVehile3DInfo输出口数据进行打包
      | //两个结构体的长度都是152
      | sizeof(SOut2Simulator) = sizeof(MavVehileInfo) = 152
      |
      | 打包封装的结构体为
      | typedef struct _netDataShort
      | {
      | TargetType tg; //这里目前随便填，写1即可 uint32
      | int len; //这个长度为传输结构体长度，目前是152
      | char payload[192]; //这里面前152位存放了SOut2Simulator结构体数据，后面的40位保留
      | }netDataShort;
      |
      | //UDP包的总长度为200
      | sizeof(netDataShort) = 200
      |
      | //发送的UDP端口号为：20010
  copterID : Inport  PortDimensions=1
  vehicleType : Inport  Port=2  PortDimensions=1
  runnedTime : Inport  Port=3  PortDimensions=1
  "VelE " : Inport  Port=4  PortDimensions=3
  PosE : Inport  Port=5  PortDimensions=3
  AngEuler : Inport  Port=6  PortDimensions=3
  AngQuatern : Inport  Port=7  PortDimensions=4
  MotorRPMS : Inport  Port=8  PortDimensions=8
  AccB : Inport  Port=9  PortDimensions=3
  RateB : Inport  Port=10  PortDimensions=3
  PosGPS : Inport  Port=11  PortDimensions=3
  Data Type Conversion : DataTypeConversion  OutDataTypeStr=uint32  SaturateOnIntegerOverflow=off  RndMeth=Floor
  Data Type Conversion1 : DataTypeConversion  OutDataTypeStr=int32  SaturateOnIntegerOverflow=off  RndMeth=Floor
  Data Type Conversion2 : DataTypeConversion  OutDataTypeStr=int32  SaturateOnIntegerOverflow=off  RndMeth=Floor
  Data Type Conversion3 : DataTypeConversion  OutDataTypeStr=int32  SaturateOnIntegerOverflow=off  RndMeth=Floor
  Data Type Conversion4 : DataTypeConversion  OutDataTypeStr=double  SaturateOnIntegerOverflow=off  RndMeth=Floor
  Data Type Conversion5 : DataTypeConversion  OutDataTypeStr=single  SaturateOnIntegerOverflow=off  RndMeth=Floor
  Data Type Conversion6 : DataTypeConversion  OutDataTypeStr=double  SaturateOnIntegerOverflow=off  RndMeth=Floor
  Data Type Conversion7 : DataTypeConversion  OutDataTypeStr=double  SaturateOnIntegerOverflow=off  RndMeth=Floor
  Mux : Mux  Inputs=2
  Mux1 : Mux  Inputs=7
  Mux2 : Mux  Inputs=2
  Package Head : etargetslib/Byte Pack  datatypes={'uint32','int32'}  byteAlign=4
  PayLoad : etargetslib/Byte Pack  datatypes={'int32','double','single','double','double'}  byteAlign=8
  TargetType : Constant  OutDataTypeStr=Inherit: Inherit via back propagation
  len : Constant  Value=152  OutDataTypeStr=Inherit: Inherit via back propagation
  reserve : Constant  Value=[0 0 0 0 0]  OutDataTypeStr=double
  toUnReal : Outport  VectorParamsAs1DForOutWhenUnconnected=off
  wires:
  runnedTime/1 -> Data Type Conversion4/1
  RateB/1 -> Mux1/7
  PayLoad/1 -> Mux/2
  "VelE "/1 -> Mux1/1
  Mux1/1 -> Data Type Conversion5/1
  PosGPS/1 -> Data Type Conversion6/1
  Package Head/1 -> Mux/1
  AccB/1 -> Mux1/6
  Mux/1 -> toUnReal/1
  MotorRPMS/1 -> Mux1/5
  AngQuatern/1 -> Mux1/4
  copterID/1 -> Data Type Conversion2/1
  len/1 -> Data Type Conversion1/1
  vehicleType/1 -> Data Type Conversion3/1
  PosE/1 -> Mux1/2
  TargetType/1 -> Data Type Conversion/1
  reserve/1 -> Data Type Conversion7/1
  Mux2/1 -> PayLoad/1
  AngEuler/1 -> Mux1/3
  Data Type Conversion5/1 -> PayLoad/3
  Data Type Conversion2/1 -> Mux2/1
  Data Type Conversion1/1 -> Package Head/2
  Data Type Conversion6/1 -> PayLoad/4
  Data Type Conversion/1 -> Package Head/1
  Data Type Conversion3/1 -> Mux2/2
  Data Type Conversion4/1 -> PayLoad/2
  Data Type Conversion7/1 -> PayLoad/5

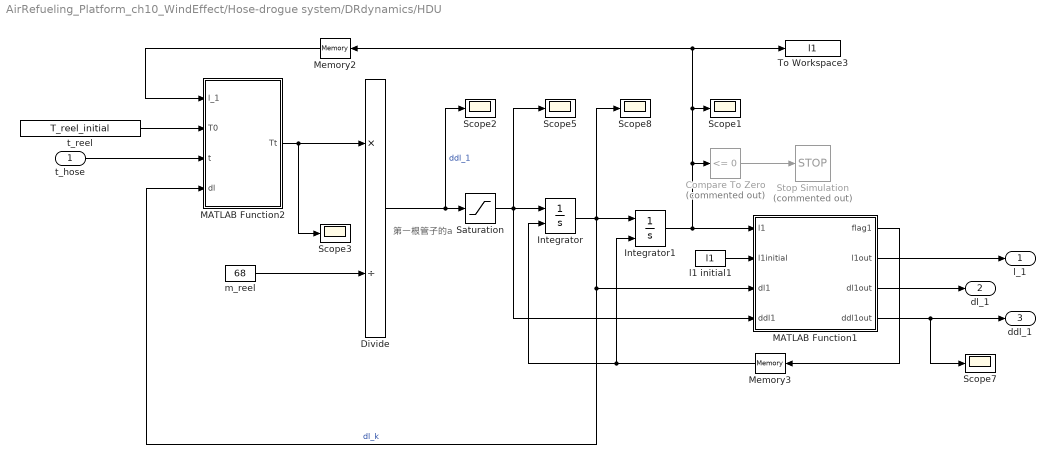
== system AirRefueling_Platform_ch10_WindEffect/Hose-drogue system/DRdynamics/HDU ==
  note: 第一根管子的a
  t_hose : Inport
  Compare To Zero : simulink/Logic and Bit Operations/Compare To Zero  Commented=on  relop=<=  OutDataTypeStr=boolean
  Divide : Product  Inputs=*/
  Integrator : Integrator  ExternalReset=rising  UpperSaturationLimit=0.3  LowerSaturationLimit=-0.3
  Integrator1 : Integrator  ExternalReset=rising  InitialCondition=l1
  MATLAB Function1 : MATLAB Function  TreatAsAtomicUnit=on
  MATLAB Function2 : MATLAB Function  TreatAsAtomicUnit=on
  Memory2 : Memory  InitialCondition=l1
  Memory3 : Memory
  Saturation : Saturate  UpperLimit=3  LowerLimit=-3
  Scope{1..3,5,7..8} (6 alike) : Scope
  Stop Simulation : Stop  Commented=on
  To Workspace3 : ToWorkspace  VariableName=l1  SampleTime=-1
  l1 initial1 : Constant  Value=l1
  m_reel : Constant  Value=68
  t_reel : Constant  Value=T_reel_initial
  l_1 : Outport
  dl_1 : Outport  Port=2
  ddl_1 : Outport  Port=3
  wires:
  MATLAB Function2/1(Tt) -> Scope3/1, Divide/1
  m_reel/1 -> Divide/2
  Divide/1 -> Saturation/1, Scope2/1  "ddl_1"
  Integrator/1 -> Integrator1/1, MATLAB Function1/3(dl1), MATLAB Function2/4(dl), Scope8/1  "dl_k"
  Saturation/1 -> MATLAB Function1/4(ddl1), Integrator/1, Scope5/1
  t_reel/1 -> MATLAB Function2/2(T0)
  Compare To Zero/1 -> Stop Simulation/1
  l1 initial1/1 -> MATLAB Function1/2(l1initial)
  MATLAB Function1/4(ddl1out) -> Scope7/1, ddl_1/1
  MATLAB Function1/1(flag1) -> Memory3/1
  Memory2/1 -> MATLAB Function2/1(l_1)
  Memory3/1 -> Integrator/2, Integrator1/2
  Integrator1/1 -> MATLAB Function1/1(l1), Compare To Zero/1, To Workspace3/1, Memory2/1, Scope1/1
  MATLAB Function1/2(l1out) -> l_1/1
  MATLAB Function1/3(dl1out) -> dl_1/1
  t_hose/1 -> MATLAB Function2/3(t)

== system AirRefueling_Platform_ch10_WindEffect/Hose-drogue system/DRdynamics/Hose-Drogue1 ==
  note: % vr = 连杆相对风速度 向量3*N
      | % n = 连杆的方向向量，向上为正 向量3*N
  note: link1的加速度
  note: tanker的加速度
  note: 3*N的数组
  note: 扰动等的力
  note: 高度生成密度和粘滞系数
  pt : Inport
  vt : Inport  Port=2
  at : Inport  Port=3
  w : Inport  Port=4
  link length : Inport  Port=5
  D link length : Inport  Port=6
  DD link length : Inport  Port=7
  Fb : Inport  Port=8
  Atmosphere Data : Subsystem
  Calculate the Acceleration of the Links1 : Subsystem
  Calculate the External Force of the Links : Subsystem
  Calculate the Orientation of the Links1 : Subsystem
  Height : Constant  Value=height
  MATLAB Function3 : MATLAB Function  TreatAsAtomicUnit=on
  Scope : Scope
  Scope1 : Scope
  Scope8 : Scope
  link line density : Constant  Value=l_density
  link radius : Constant  Value=Rl
  p link : Outport
  t : Outport  Port=2
  pdr : Outport  Port=3
  wires:
  Height/1 -> Atmosphere Data/1(height)
  Atmosphere Data/1(densitiy) -> Calculate the External Force of the Links/6(density)
  Atmosphere Data/2(viscosity) -> Calculate the External Force of the Links/7(viscosity)
  link radius/1 -> Calculate the External Force of the Links/4(link radius)
  link line density/1 -> Calculate the External Force of the Links/5(link line density), Calculate the Acceleration of the Links1/5(link line density)
  Calculate the External Force of the Links/1(Q) -> Scope/1, Calculate the Acceleration of the Links1/1(Q)
  Calculate the Orientation of the Links1/1(n) -> Calculate the External Force of the Links/2(n), MATLAB Function3/1(n), Calculate the Acceleration of the Links1/3(n)
  Calculate the Orientation of the Links1/2(dn) -> Calculate the Acceleration of the Links1/4(dn)
  Calculate the External Force of the Links/2(Mdr) -> Calculate the Acceleration of the Links1/2(Mdr)
  at/1 -> Calculate the Orientation of the Links1/4(at), Calculate the Acceleration of the Links1/8("tanker acceleration ")
  Calculate the Orientation of the Links1/3(vr) -> Calculate the External Force of the Links/1(vr)
  w/1 -> Calculate the Orientation of the Links1/6(w)
  Calculate the Acceleration of the Links1/1(a) -> Calculate the Orientation of the Links1/3(a), Scope8/1
  Calculate the Orientation of the Links1/4(p) -> Calculate the External Force of the Links/8(p), p link/1
  pt/1 -> Calculate the Orientation of the Links1/7(pt)
  vt/1 -> Calculate the Orientation of the Links1/5(vt)
  Calculate the Acceleration of the Links1/2(t) -> t/1
  link length/1 -> Calculate the Orientation of the Links1/1(link length), Calculate the External Force of the Links/3(l1), Calculate the Acceleration of the Links1/6(l1 length)
  D link length/1 -> Calculate the Orientation of the Links1/2(D link length)
  DD link length/1 -> Calculate the Acceleration of the Links1/7(DD l1 length)
  Fb/1 -> Calculate the External Force of the Links/9(Fb)
  MATLAB Function3/1(alpha) -> Scope1/1
  Calculate the Orientation of the Links1/5(pdr) -> pdr/1

== system AirRefueling_Platform_ch10_WindEffect/Receiver system/F16 Nonlinear Model/Adding Wind Disturbance ==
  Speed of Sound : Inport
  Air Density : Inport  Port=2
  Wind Velocity : Inport  Port=3  PortDimensions=3
  Wind Angular Rates : Inport  Port=4  PortDimensions=3
  Vb : Inport  Port=5  PortDimensions=3
  p,q,r : Inport  Port=6  PortDimensions=3
  Dynamic Pressure : aerolibasang/Dynamic Pressure
  "Incidence, Sideslip & Airspeed" : aerolibasang/Incidence, Sideslip, & Airspeed
  Mach Number : aerolibasang/Mach Number
      settings: SourceProductBaseCode=AE
  Mux : Mux  Inputs=2
  Sum : Sum  Inputs=|+-  InputSameDT=on  SaturateOnIntegerOverflow=on  OutDataTypeStr=Inherit: Same as first input
  Sum1 : Sum  Inputs=|++  InputSameDT=on  SaturateOnIntegerOverflow=on  OutDataTypeStr=Inherit: Same as first input
  qbar : Outport  InitialOutput=0
  "p,q,r " : Outport  Port=2
  V : Outport  Port=3
  Mach : Outport  Port=4
  Incid : Outport  Port=5
  wires:
  "Incidence, Sideslip & Airspeed"/3 -> V/1
  Dynamic Pressure/1 -> qbar/1
  Air Density/1 -> Dynamic Pressure/2
  Mach Number/1 -> Mach/1
  Sum/1 -> Dynamic Pressure/1, Mach Number/1, "Incidence, Sideslip & Airspeed"/1
  Vb/1 -> Sum/1
  Speed of Sound/1 -> Mach Number/2
  Wind Velocity/1 -> Sum/2
  "Incidence, Sideslip & Airspeed"/2 -> Mux/2  "Beta"
  Mux/1 -> Incid/1
  "Incidence, Sideslip & Airspeed"/1 -> Mux/1  "Alpha"
  p,q,r/1 -> Sum1/1
  Wind Angular Rates/1 -> Sum1/2
  Sum1/1 -> "p,q,r "/1

== system AirRefueling_Platform_ch10_WindEffect/Receiver system/F16 Nonlinear Model/Aerodynamic Coefficients ==
  Actuators : Inport
  Incid : Inport  Port=2
  Mach : Inport  Port=3
  V : Inport  Port=4
  p,q,r : Inport  Port=5
  qbar/ps : Inport  Port=6
  Angle Conversion : aerolibconvert2/Angle Conversion  IU=rad  OU=deg
  Interpreted MATLAB Function : MATLABFcn  MATLABFcn=F16Coef1  OutputDimensions=6
  Leading Edge Flap : Subsystem
  Mux : Mux  Inputs=6
  Terminator2 : Terminator
  alpha : Selector  InputPortWidth=2  IndexOptions=Index vector (dialog)  Indices=1  OutputSizes=1
  flag : Constant  Value=fi_flag
  Coeff : Outport  InitialOutput=0
  wires:
  Angle Conversion/1 -> alpha/1, Mux/2
  Incid/1 -> Angle Conversion/1
  qbar/ps/1 -> Leading Edge Flap/2(qbar/ps)
  alpha/1 -> Leading Edge Flap/1(alpha)
  V/1 -> Mux/1
  p,q,r/1 -> Mux/3
  Actuators/1 -> Mux/4
  flag/1 -> Mux/5
  Mach/1 -> Terminator2/1
  Interpreted MATLAB Function/1 -> Coeff/1
  Mux/1 -> Interpreted MATLAB Function/1
  Leading Edge Flap/1(delta_lef (deg)) -> Mux/6

== system AirRefueling_Platform_ch10_WindEffect/Receiver system/F16 Nonlinear Model/Environment Models ==
  Xe : Inport  PortDimensions=3
  DCM : Inport  Port=2
  COESA Atmosphere Model : aerolibatmos2/COESA Atmosphere Model  units=English (Velocity in ft/s)  spec=1976 COESA-extended U.S. Standard Atmosphere  model=Profile  profile_var=High temperature  profile_percent=10%  profile_alt=5 km (16404 ft)  envelope_var=High temperature  envelope_percent=1%  action=None
  Gravity in Earth Axes : Gain  Gain=mass  SaturateOnIntegerOverflow=on  OutDataTypeStr=Inherit: Same as input  ParamDataTypeStr=Inherit: Same as input
  Height : Selector  InputPortWidth=3  IndexOptions=Index vector (dialog)  Indices=[3]  OutputSizes=1
  Inertial to Body : Product  Multiplication=Matrix(*)  InputSameDT=on  SaturateOnIntegerOverflow=on  OutDataTypeStr=Inherit: Same as first input
  Latitude : Constant  Value=0
  Mux : Mux  Inputs=3
  Product6 : Product  Inputs=**  InputSameDT=on  SaturateOnIntegerOverflow=on  OutDataTypeStr=Inherit: Same as first input
  Reshape : Reshape
  Terminator : Terminator
  "WGS84 Gravity Model " : aerolibobsolete/WGS84 Gravity Model   model=WGS84 Taylor Series  units=English  no_atmos=on  precessing=on  jd_loc=off  month=October  day=10  year=2004  no_centrifugal=on  action=None
      settings: SourceProductBaseCode=AE
  r2d5 : Gain  Gain=1715  SaturateOnIntegerOverflow=on  OutDataTypeStr=Inherit: Same as input  ParamDataTypeStr=Inherit: Same as input
  z-->h : Abs
  Fg : Outport  InitialOutput=0
  Speed of Sound : Outport  Port=2  InitialOutput=0
  Air Density : Outport  Port=3  InitialOutput=0
  PS : Outport  Port=4
  wires:
  Reshape/1 -> Inertial to Body/2
  Mux/1 -> "WGS84 Gravity Model "/1
  z-->h/1 -> Mux/3, COESA Atmosphere Model/1
  COESA Atmosphere Model/2 -> Speed of Sound/1
  COESA Atmosphere Model/3 -> Terminator/1
  Height/1 -> z-->h/1
  Xe/1 -> Height/1
  Latitude/1 -> Mux/2, Mux/1
  "WGS84 Gravity Model "/1 -> Gravity in Earth Axes/1
  Gravity in Earth Axes/1 -> Reshape/1
  DCM/1 -> Inertial to Body/1
  Inertial to Body/1 -> Fg/1
  COESA Atmosphere Model/4 -> Product6/2, Air Density/1
  COESA Atmosphere Model/1 -> r2d5/1
  Product6/1 -> PS/1
  r2d5/1 -> Product6/1

== system AirRefueling_Platform_ch10_WindEffect/Receiver system/F16 Nonlinear Model/Forces and Moments ==
  Coeff : Inport
  Thrust : Inport  Port=2
  qbar : Inport  Port=3
  "Aerodynamic Forces and Moments " : aerolibadyn/Aerodynamic Forces and Moments   inputAxes=Body  outputForceAxes=Body  outputMomentAxes=Body  S=S_ref  b=b_ref  cbar=d_ref
  Center of Gravity : Constant  Value=[-0 0 0]
  Center of Pressure : Constant  Value=[-0 0 0]
  Sum : Sum  Inputs=++|  InputSameDT=on  SaturateOnIntegerOverflow=on  OutDataTypeStr=Inherit: Same as first input
  X,Y,Z : Outport  InitialOutput=0
  LMN : Outport  Port=2  InitialOutput=0
  wires:
  Center of Pressure/1 -> "Aerodynamic Forces and Moments "/4
  Center of Gravity/1 -> "Aerodynamic Forces and Moments "/3
  "Aerodynamic Forces and Moments "/1 -> Sum/2
  "Aerodynamic Forces and Moments "/2 -> LMN/1
  Sum/1 -> X,Y,Z/1
  Thrust/1 -> Sum/1
  qbar/1 -> "Aerodynamic Forces and Moments "/2
  Coeff/1 -> "Aerodynamic Forces and Moments "/1
